simulink model "Base_Map_M_cs"  (R2017b)
settings: Solver=FixedStepDiscrete  StartTime=0.0  StopTime=60  FixedStep=1/100  RelTol=1e-3
PreLoadFcn:
  | mbxruntime.callbacks.PreLoadFcn(bdroot);
  | check_NUTS_defined
  | model_closed = 0;
  | assignin('base',['model_closed_' bdroot],false);
PostLoadFcn:
  | mbxruntime.callbacks.PostLoadFcn(bdroot);
InitFcn:
  | mbxruntime.callbacks.InitFcn(bdroot);
StartFcn:
  | mbxruntime.callbacks.StartFcn(bdroot);
StopFcn:
  | mbxruntime.callbacks.StopFcn(bdroot);;
  | 
model workspace: external: MAT-File Base_Map_M_cs_hws.mat (data not in the file)
undefined symbols (not defined in the file): mbxruntime, tabledata
(part 1 of 3)
CloseFcn:
  | mbxruntime.callbacks.CloseFcn(bdroot);
  | evalin('base',['clear model_closed_' bdroot]);
  | model_closed = 1;
settings Model: Creator=PRESCAN  LastModifiedBy=naveenm
settings DataIOCC: LimitDataPoints=on  SaveFormat=Array  SignalLoggingSaveFormat=ModelDataLogs
settings OptimizationCC: ExpressionDepthLimit=2147483647  InitFltsAndDblsToZero=on  LifeSpan=inf
settings DebuggingCC: SaveWithParameterizedLinksMsg=none  UnderspecifiedInitializationDetection=Classic  MergeDetectMultiDrivingBlocksExec=none  SignalResolutionControl=TryResolveAllWithWarning  MultiTaskDSMMsg=warning  MultiTaskCondExecSysMsg=none  FcnCallInpInsideContextMsg=warning  StateNameClashWarn=warning  SFUnexpectedBacktrackingDiag=warning  SFNoUnconditionalDefaultTransitionDiag=warning  SFExecutionAtInitializationDiag=none
settings HardwareCC: ProdBitPerPointer=32  ProdBitPerSizeT=32  ProdBitPerPtrDiffT=32  ProdLargestAtomicFloat=None  ProdIntDivRoundTo=Undefined  ProdEndianess=Unspecified  ProdWordSize=32  ProdHWDeviceType=32-bit Generic
settings ModelReferenceCC: UpdateModelReferenceTargets=IfOutOfDate  PropagateSignalLabelsOutOfModel=off
settings SFSimCC: SimParseCustomCode=off
settings SFSimCC: SimCustomHeaderCode=|
  | #include "prescan.h"
  | #include "prescan_platform.h"
settings CodeAppCC: StateflowObjectComments=on
settings GRTTargetCC: TargetFcnLib=ansi_tfl_tmw.mat  TargetLangStandard=C89/C90 (ANSI)  GeneratePreprocessorConditionals=Disable all  CombineOutputUpdateFcns=off  GRTInterface=on
settings ConfigComp: CovMetricSettings=dw  CovHtmlReporting=on  CovSaveCumulativeToWorkspaceVar=on  CovSaveSingleToWorkspaceVar=on  CovExternalEMLEnable=off

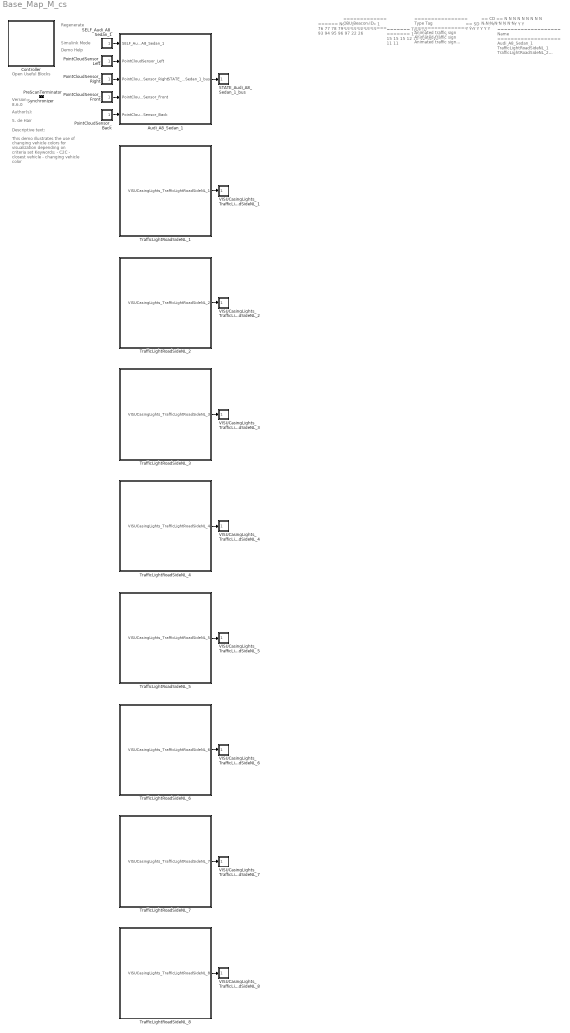
== system Base_Map_M_cs ==
  note: Regenerate
  note: Simulink Mode
  note: Open Useful Blocks
  note: 8.6.0
  note: Version:
  note: Author(s):
  note: S. de Hair
  note: Descriptive text:
  note: This demo illustrates the use of
      | changing vehicle colors for
      | visualization depending on
      | criteria set
      |
      |
      |
      | Keywords:
      |
      | - C2C
      |
      | - closest vehicle
      |
      | - changing vehicle color
  note: Demo Help
  note: ======
      | Num ID
      | ======
      | 1
      | 76
      | 77
      | 78
      | 79
      | 80
      | 81
      | 82
      | 83
      | 91
      | 93
      | 94
      | 95
      | 96
      | 97
      | 22
      | 26
  note: =============
      | OBU-Beacon ID
      | =============
  note: =======
      | Type ID
      | =======
      | 1
      | 15
      | 15
      | 15
      | 15
      | 15
      | 15
      | 15
      | 15
      | 12
      | 12
      | 12
      | 12
      | 12
      | 12
      | 11
      | 11
  note: ================
      | Type Tag
      | ================
      | Car
      | Animated traffic sign
      | Animated traffic sign
      | Animated traffic sign
      | Animated traffic sign
      | Animated traffic sign
      | Animated traffic sign
      | Animated traffic sign
      | Animated traffic sign
      | Building
      | Building
      | Building
      | Building
      | Building
      | Building
      | Road
      | Road
  note: ==
      | SD
      | ==
      | Y
      | Y
      | Y
      | Y
      | Y
      | Y
      | Y
      | Y
      | Y
      | Y
      | Y
      | Y
      | Y
      | Y
      | Y
      | Y
      | Y
  note: ==
      | CD
      | ==
      | N
      | N
      | N
      | N
      | N
      | N
      | N
      | N
      | N
      | N
      | N
      | N
      | N
      | N
      | N
      | N
      | N
  note: ===================
      | Name
      | ===================
      | Audi_A8_Sedan_1
      | TrafficLightRoadSideNL_1
      | TrafficLightRoadSideNL_2
      | TrafficLightRoadSideNL_3
      | TrafficLightRoadSideNL_4
      | TrafficLightRoadSideNL_5
      | TrafficLightRoadSideNL_6
      | TrafficLightRoadSideNL_7
      | TrafficLightRoadSideNL_8
      | HouseOld3_1
      | HouseOld4_1
      | HouseOld5_1
      | School_1
      | OfficeBrownFlat_1
      | OfficeBrownTall2_1
      | StraightRoad_2
      | StraightRoad_5
  Audi_A8_Sedan_1 : Subsystem  Tag=WorldObjectSubSystem  InitFcn=UniqueId = '642';
      mask init:
      | modelPath = GenericModelHelper.getGenericModelFilePath('ModelDepo','Vehicles\Audi_A8\Audi_A8.pgmb','d771622804618130053427da08a6d484');imagePath = GenericModelHelper.getCompilationPicture(modelPath, 'Audi_A8_HighPoly.png');
      mask Display: image(imread(imagePath));color('white');text(0, 0, ' ID=1\n')
  Controller : Subsystem  Description=6E19BCF7C30917F51270F1088431415395D17B111411129AD7F824A4489CC94F  Priority=-1  LoadFcn=load PreScanControllerData  mask(PreScan Simulation Controller){prescanversion='8.6.0', ModelReferencing=off, TimeStep=1/100, ControlMode=0, PreScanExecutionMode=on, ControllerCount=0, ControllerIndex=0, ControllerOptions=''}
      mask prompts: prescanversion "PreScan Version"; ModelReferencing "Use Model Referencing"; TimeStep "Upload Period [s]"; ControlMode "Control Mode"; PreScanExecutionMode "Execution Mode"; ControllerCount "Controller Count"; ControllerIndex "Controller Index"; ControllerOptions "Controller Options"
      mask help:
      | Please do not remove this block from the compilation sheet,
      | as it connects the model to the PreScan environment.
      mask init:
      | model = bdroot(gcb);
      | ExperimentFile = mbxruntime.findExperimentFile(model,true); %relative path
      | 
      | [d1, d2, d3, prescandata] = prescan_Settings();
      | ModelDepo = fullfile(prescandata,'ModelDepo'); 
      | 
      | RTmode = mbxruntime.getRTMode(model);
      | 
      | SimulationMode = get_param(bdroot,'SimulationMode');
      | if strcmp(SimulationMode, 'rapid-accelerator')
      |     SimulationMode = 'external';
      | end
      | TargetName = get_param(bdroot,'SystemTargetFile');
      settings: ModelCloseFcn=assignin('base',['model_closed_' bdroot],true);
      mask Help: eval('openHelp(812)')
      mask Display: image(imread('prescanlogo.ico'))
  PointCloudSensor_Back : Subsystem  Tag=sensor/PointCloudInport  Priority=3  mask(PreScan Source Block: Point Cloud Sensor){}
      mask help: The Point Cloud Sensor provides XYZ positions relative to the sensor
      settings: OpenFcn=open_system([gcb '/Sensor'],'mask')
      mask Help: eval('openHelp(6400)')
      mask Display: image(imread('PointCloudSensorSL.png'))
  PointCloudSensor_Front : Subsystem  Tag=sensor/PointCloudInport  Priority=3  mask(PreScan Source Block: Point Cloud Sensor){}
      mask help: The Point Cloud Sensor provides XYZ positions relative to the sensor
      settings: OpenFcn=open_system([gcb '/Sensor'],'mask')
      mask Help: eval('openHelp(6400)')
      mask Display: image(imread('PointCloudSensorSL.png'))
  PointCloudSensor_Left : Subsystem  Tag=sensor/PointCloudInport  Priority=3  mask(PreScan Source Block: Point Cloud Sensor){}
      mask help: The Point Cloud Sensor provides XYZ positions relative to the sensor
      settings: OpenFcn=open_system([gcb '/Sensor'],'mask')
      mask Help: eval('openHelp(6400)')
      mask Display: image(imread('PointCloudSensorSL.png'))
  PointCloudSensor_Right : Subsystem  Tag=sensor/PointCloudInport  Priority=3  mask(PreScan Source Block: Point Cloud Sensor){}
      mask help: The Point Cloud Sensor provides XYZ positions relative to the sensor
      settings: OpenFcn=open_system([gcb '/Sensor'],'mask')
      mask Help: eval('openHelp(6400)')
      mask Display: image(imread('PointCloudSensorSL.png'))
  PreScanTerminator : Subsystem  Tag=PreScanTerminator  Priority=999  LoadFcn=load PrescanTerminatorData  mask(PreScan Simulation Terminator){TimeStep=1/100}
      mask prompts: TimeStep "Upload Period [s]"
      mask help:
      | Please do not remove this block from the compilation sheet as it
      | connects the model to the PreScan environment.
      mask Help: eval('openHelp(812)')
      mask Display: image(imread('prescanlogo.ico'))
  SELF_Audi_A8_Sedan_1 : Subsystem  Tag=sensor/SelfPort  Priority=3  LoadFcn=load('PreScanSelfSensorData.mat')  mask(PreScan Source Block: SELF){}
      mask help:
      | The SELF port shows (state) information of the actor itself. The outputs are position in the experiment's axis system and the GPS coordinates, and the object's absolute velocity and compass heading.
      |
      | For more information, please click Help.
      settings: OpenFcn=open_system([gcb '/Sensor'],'mask')
      mask Help: eval('openHelp(462)')
      mask Display: image(imread('GPS.png'))
  STATE_Audi_A8_Sedan_1_bus : Subsystem  Tag=actuator/StatePort  Priority=0  LoadFcn=load('PreScanStateActuatorData.mat')  mask(PreScan Sink Block: State){}
      mask help:
      | The Actor State contains a vector signal of size (9x1), containing the following signals:
      |
      | -  Position    	(x,y,z)             	[m]
      | -  Velocity    	(vx,vy,vz)         	[m/s]
      | -  Angles       	(Roll, Pitch, Yaw)	[rad]
      |
      | The Actor state is defined in the global axis system.
      | The state is superponed on the Initial position defined in the GUI.
      |
      | For more information, please click Help.
      settings: OpenFcn=open_system([gcb '/Actuator'],'mask')
      mask Help: eval('openHelp(222)')
      mask Display: image(imread('State.png'))
  Synchronizer : Subsystem  Tag=PreScanSynchronizer  Priority=1  LoadFcn=load PrescanSynchronizeData  mask(PreScan Simulation Core Block){TimeStep=1/100}
      mask prompts: TimeStep "Timestep [s]"
      mask help:
      | Please do not remove this block from the PreScan compilation sheet,
      | as it contains essential configuration parameters for a PreScan simulation.
      settings: DeleteFcn=PreScanBlockDeleteFcn;
      mask Display: image(imread('prescanlogo.ico'))
  TrafficLightRoadSideNL_1 : Subsystem  Tag=WorldObjectSubSystem  InitFcn=UniqueId = '646';
      mask init:
      | imagePath=which('TrafficLightRoadSideNL.jpg');
      mask Display: image(imread(imagePath));color('white');text(0, 0, ' ID=76\n')
  TrafficLightRoadSideNL_2 : Subsystem  Tag=WorldObjectSubSystem  InitFcn=UniqueId = '647';
      mask init:
      | imagePath=which('TrafficLightRoadSideNL.jpg');
      mask Display: image(imread(imagePath));color('white');text(0, 0, ' ID=77\n')
  TrafficLightRoadSideNL_3 : Subsystem  Tag=WorldObjectSubSystem  InitFcn=UniqueId = '649';
      mask init:
      | imagePath=which('TrafficLightRoadSideNL.jpg');
      mask Display: image(imread(imagePath));color('white');text(0, 0, ' ID=78\n')
  TrafficLightRoadSideNL_4 : Subsystem  Tag=WorldObjectSubSystem  InitFcn=UniqueId = '650';
      mask init:
      | imagePath=which('TrafficLightRoadSideNL.jpg');
      mask Display: image(imread(imagePath));color('white');text(0, 0, ' ID=79\n')
  TrafficLightRoadSideNL_5 : Subsystem  Tag=WorldObjectSubSystem  InitFcn=UniqueId = '651';
      mask init:
      | imagePath=which('TrafficLightRoadSideNL.jpg');
      mask Display: image(imread(imagePath));color('white');text(0, 0, ' ID=80\n')
  TrafficLightRoadSideNL_6 : Subsystem  Tag=WorldObjectSubSystem  InitFcn=UniqueId = '652';
      mask init:
      | imagePath=which('TrafficLightRoadSideNL.jpg');
      mask Display: image(imread(imagePath));color('white');text(0, 0, ' ID=81\n')
  TrafficLightRoadSideNL_7 : Subsystem  Tag=WorldObjectSubSystem  InitFcn=UniqueId = '653';
      mask init:
      | imagePath=which('TrafficLightRoadSideNL.jpg');
      mask Display: image(imread(imagePath));color('white');text(0, 0, ' ID=82\n')
  TrafficLightRoadSideNL_8 : Subsystem  Tag=WorldObjectSubSystem  InitFcn=UniqueId = '654';
      mask init:
      | imagePath=which('TrafficLightRoadSideNL.jpg');
      mask Display: image(imread(imagePath));color('white');text(0, 0, ' ID=83\n')
  VISUCasingLights_TrafficLightRoadSideNL_1 : Subsystem  Tag=actuator/VisuCasingLights  Priority=0  mask(PreScan Sink Block: VisuTrafficLight){UniqueID=646, ColorsObjectQuery=, Colors=[]}
      mask prompts: UniqueID "Parent Unique Identifier"; ColorsObjectQuery "Query for Color Object"; Colors "Matrix of colors"
      mask help:
      | The VisuTrafficLight block provides a way to animate traffic lights: switch on and off individual lights.
      |
      | For more information, please click Help.
      settings: OpenFcn=open_system([gcb '/Actuator'],'mask')
      mask Help: eval('openHelp(731)')
      mask Display: image(imread('TrafficLightCasing.png'))
  VISUCasingLights_TrafficLightRoadSideNL_2 : Subsystem  Tag=actuator/VisuCasingLights  Priority=0  mask(PreScan Sink Block: VisuTrafficLight){UniqueID=647, ColorsObjectQuery=, Colors=[]}
      mask prompts: UniqueID "Parent Unique Identifier"; ColorsObjectQuery "Query for Color Object"; Colors "Matrix of colors"
      mask help:
      | The VisuTrafficLight block provides a way to animate traffic lights: switch on and off individual lights.
      |
      | For more information, please click Help.
      settings: OpenFcn=open_system([gcb '/Actuator'],'mask')
      mask Help: eval('openHelp(731)')
      mask Display: image(imread('TrafficLightCasing.png'))
  VISUCasingLights_TrafficLightRoadSideNL_3 : Subsystem  Tag=actuator/VisuCasingLights  Priority=0  mask(PreScan Sink Block: VisuTrafficLight){UniqueID=649, ColorsObjectQuery=, Colors=[]}
      mask prompts: UniqueID "Parent Unique Identifier"; ColorsObjectQuery "Query for Color Object"; Colors "Matrix of colors"
      mask help:
      | The VisuTrafficLight block provides a way to animate traffic lights: switch on and off individual lights.
      |
      | For more information, please click Help.
      settings: OpenFcn=open_system([gcb '/Actuator'],'mask')
      mask Help: eval('openHelp(731)')
      mask Display: image(imread('TrafficLightCasing.png'))
  VISUCasingLights_TrafficLightRoadSideNL_4 : Subsystem  Tag=actuator/VisuCasingLights  Priority=0  mask(PreScan Sink Block: VisuTrafficLight){UniqueID=650, ColorsObjectQuery=, Colors=[]}
      mask prompts: UniqueID "Parent Unique Identifier"; ColorsObjectQuery "Query for Color Object"; Colors "Matrix of colors"
      mask help:
      | The VisuTrafficLight block provides a way to animate traffic lights: switch on and off individual lights.
      |
      | For more information, please click Help.
      settings: OpenFcn=open_system([gcb '/Actuator'],'mask')
      mask Help: eval('openHelp(731)')
      mask Display: image(imread('TrafficLightCasing.png'))
  VISUCasingLights_TrafficLightRoadSideNL_5 : Subsystem  Tag=actuator/VisuCasingLights  Priority=0  mask(PreScan Sink Block: VisuTrafficLight){UniqueID=651, ColorsObjectQuery=, Colors=[]}
      mask prompts: UniqueID "Parent Unique Identifier"; ColorsObjectQuery "Query for Color Object"; Colors "Matrix of colors"
      mask help:
      | The VisuTrafficLight block provides a way to animate traffic lights: switch on and off individual lights.
      |
      | For more information, please click Help.
      settings: OpenFcn=open_system([gcb '/Actuator'],'mask')
      mask Help: eval('openHelp(731)')
      mask Display: image(imread('TrafficLightCasing.png'))
  VISUCasingLights_TrafficLightRoadSideNL_6 : Subsystem  Tag=actuator/VisuCasingLights  Priority=0  mask(PreScan Sink Block: VisuTrafficLight){UniqueID=652, ColorsObjectQuery=, Colors=[]}
      mask prompts: UniqueID "Parent Unique Identifier"; ColorsObjectQuery "Query for Color Object"; Colors "Matrix of colors"
      mask help:
      | The VisuTrafficLight block provides a way to animate traffic lights: switch on and off individual lights.
      |
      | For more information, please click Help.
      settings: OpenFcn=open_system([gcb '/Actuator'],'mask')
      mask Help: eval('openHelp(731)')
      mask Display: image(imread('TrafficLightCasing.png'))
  VISUCasingLights_TrafficLightRoadSideNL_7 : Subsystem  Tag=actuator/VisuCasingLights  Priority=0  mask(PreScan Sink Block: VisuTrafficLight){UniqueID=653, ColorsObjectQuery=, Colors=[]}
      mask prompts: UniqueID "Parent Unique Identifier"; ColorsObjectQuery "Query for Color Object"; Colors "Matrix of colors"
      mask help:
      | The VisuTrafficLight block provides a way to animate traffic lights: switch on and off individual lights.
      |
      | For more information, please click Help.
      settings: OpenFcn=open_system([gcb '/Actuator'],'mask')
      mask Help: eval('openHelp(731)')
      mask Display: image(imread('TrafficLightCasing.png'))
  VISUCasingLights_TrafficLightRoadSideNL_8 : Subsystem  Tag=actuator/VisuCasingLights  Priority=0  mask(PreScan Sink Block: VisuTrafficLight){UniqueID=654, ColorsObjectQuery=, Colors=[]}
      mask prompts: UniqueID "Parent Unique Identifier"; ColorsObjectQuery "Query for Color Object"; Colors "Matrix of colors"
      mask help:
      | The VisuTrafficLight block provides a way to animate traffic lights: switch on and off individual lights.
      |
      | For more information, please click Help.
      settings: OpenFcn=open_system([gcb '/Actuator'],'mask')
      mask Help: eval('openHelp(731)')
      mask Display: image(imread('TrafficLightCasing.png'))
  wires:
  Audi_A8_Sedan_1/1(STATE_Audi_A8_Sedan_1_bus) -> STATE_Audi_A8_Sedan_1_bus/1(STATE_Audi_A8_Sedan_1_bus)
  SELF_Audi_A8_Sedan_1/1(SELF_Audi_A8_Sedan_1) -> Audi_A8_Sedan_1/1(SELF_Audi_A8_Sedan_1)
  PointCloudSensor_Left/1(PointCloudSensor_Left) -> Audi_A8_Sedan_1/2(PointCloudSensor_Left)
  PointCloudSensor_Right/1(PointCloudSensor_Right) -> Audi_A8_Sedan_1/3(PointCloudSensor_Right)
  PointCloudSensor_Front/1(PointCloudSensor_Front) -> Audi_A8_Sedan_1/4(PointCloudSensor_Front)
  PointCloudSensor_Back/1(PointCloudSensor_Back) -> Audi_A8_Sedan_1/5(PointCloudSensor_Back)
  TrafficLightRoadSideNL_1/1(VISUCasingLights_TrafficLightRoadSideNL_1) -> VISUCasingLights_TrafficLightRoadSideNL_1/1(VISUCasingLights_TrafficLightRoadSideNL_1)
  TrafficLightRoadSideNL_2/1(VISUCasingLights_TrafficLightRoadSideNL_2) -> VISUCasingLights_TrafficLightRoadSideNL_2/1(VISUCasingLights_TrafficLightRoadSideNL_2)
  TrafficLightRoadSideNL_3/1(VISUCasingLights_TrafficLightRoadSideNL_3) -> VISUCasingLights_TrafficLightRoadSideNL_3/1(VISUCasingLights_TrafficLightRoadSideNL_3)
  TrafficLightRoadSideNL_4/1(VISUCasingLights_TrafficLightRoadSideNL_4) -> VISUCasingLights_TrafficLightRoadSideNL_4/1(VISUCasingLights_TrafficLightRoadSideNL_4)
  TrafficLightRoadSideNL_5/1(VISUCasingLights_TrafficLightRoadSideNL_5) -> VISUCasingLights_TrafficLightRoadSideNL_5/1(VISUCasingLights_TrafficLightRoadSideNL_5)
  TrafficLightRoadSideNL_6/1(VISUCasingLights_TrafficLightRoadSideNL_6) -> VISUCasingLights_TrafficLightRoadSideNL_6/1(VISUCasingLights_TrafficLightRoadSideNL_6)
  TrafficLightRoadSideNL_7/1(VISUCasingLights_TrafficLightRoadSideNL_7) -> VISUCasingLights_TrafficLightRoadSideNL_7/1(VISUCasingLights_TrafficLightRoadSideNL_7)
  TrafficLightRoadSideNL_8/1(VISUCasingLights_TrafficLightRoadSideNL_8) -> VISUCasingLights_TrafficLightRoadSideNL_8/1(VISUCasingLights_TrafficLightRoadSideNL_8)

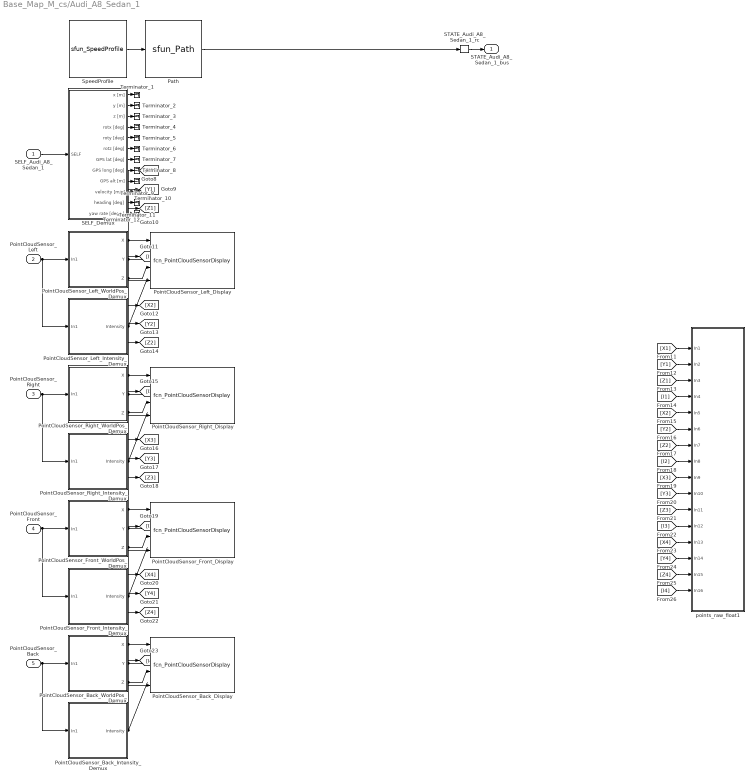
== system Base_Map_M_cs/Audi_A8_Sedan_1 ==
  SELF_Audi_A8_Sedan_1 : Inport  Tag=inport/SelfPort  OutDataTypeStr=Bus: PRESCAN_SELFSENSORDATA  PortDimensions=1  SampleTime=1/100  BusOutputAsStruct=on
  PointCloudSensor_Left : Inport  Tag=inport/PointCloudInport  Port=2  OutDataTypeStr=single  SampleTime=1/1  BusOutputAsStruct=on
  PointCloudSensor_Right : Inport  Tag=inport/PointCloudInport  Port=3  OutDataTypeStr=single  SampleTime=1/1  BusOutputAsStruct=on
  PointCloudSensor_Front : Inport  Tag=inport/PointCloudInport  Port=4  OutDataTypeStr=single  SampleTime=1/1  BusOutputAsStruct=on
  PointCloudSensor_Back : Inport  Tag=inport/PointCloudInport  Port=5  OutDataTypeStr=single  SampleTime=1/1  BusOutputAsStruct=on
  Path : S-Function  Tag=Path  LoadFcn=load('PrescanMotionData.mat')  FunctionName=sfun_Path  Parameters=uniqueID, pathUniqueID, timestep  SFunctionDeploymentMode=off  EnableBusSupport=off  mask(Path){uniqueID=642, pathUniqueID=7771, timestep=1/100}
      mask prompts: uniqueID "Object Unique ID"; pathUniqueID "Path Unique ID"; timestep "MATLAB timestep:"
      mask help:
      | The path block outputs the position along a given trajectory.
      |
      | For more information, please click Help.
      mask Help: eval('openHelp(312)')
      mask Display: image(imread('Path.png'))
  PointCloudSensor_Back_Display : M-S-Function  Tag=PointCloudSensor_Display  FunctionName=fcn_PointCloudSensorDisplay  Parameters=SensorName EnableDisplay FigureHandle EnableIntensity  mask(PreScan Point Cloud Display Block){SensorName=PointCloudSensor_Back, EnableDisplay=off, FigureHandle=64204, EnableIntensity=on}
      mask prompts: SensorName "User Specified: Title of Display"; EnableDisplay "Active"; FigureHandle "Unique Handle"; EnableIntensity "Visualize Intensity"
      mask help: This block displays world position (and intensity) output of a PreScan point cloud sensor.
      mask init:
      | if EnableDisplay
      |     EnableString='';
      |     EnableColor='gray';
      | else
      |     EnableString='INACTIVE';
      |     EnableColor='red';
      | end
      settings: DeleteFcn=PreScanBlockDeleteFcn;  ModelCloseFcn=fcn_ImageDisplay_ModelCloseFcn
      mask Help: eval('openHelp(6400)')
      mask Display:
      | color(EnableColor);
      | fprintf('%s\n PointCloud Display:\n %s',EnableString,SensorName)
      | port_label('input',1,'X')
      | port_label('input',2,'Y')
      | port_label('input',3,'Z')
      | 
      | if EnableIntensity
      |     port_label('input',4,'I')
      | end
  PointCloudSensor_Back_Intensity_Demux : Subsystem  Tag=demux/PCS/Intensity  mask{SensorName=PointCloudSensor_Back, offset=480, hres=160, vres=40}
      mask prompts: SensorName "Sensor Name"; offset "Data Start"; hres "Horizontal Resolution"; vres "Vertical Resolution"
      mask Help: eval('openHelp(6400)')
      mask Display:
      | fprintf('Point Cloud:\n Data\n %s \n %d x %d px',SensorName,hres,vres)
      | port_label('output',1,'Intensity')
  PointCloudSensor_Back_WorldPos_Demux : Subsystem  Tag=demux/PCS/WorldPos  mask{SensorName=PointCloudSensor_Back, offset=0, hres=160, vres=40}
      mask prompts: SensorName "Sensor Name"; offset "Data Start"; hres "Horizontal Resolution"; vres "Vertical Resolution"
      mask Help: eval('openHelp(6400)')
      mask Display:
      | fprintf('Point Cloud:\n Data\n %s \n %d x %d px',SensorName,hres,vres)
      | port_label('output',1,'X')
      | port_label('output',2,'Y')
      | port_label('output',3,'Z')
  PointCloudSensor_Front_Display : M-S-Function  Tag=PointCloudSensor_Display  FunctionName=fcn_PointCloudSensorDisplay  Parameters=SensorName EnableDisplay FigureHandle EnableIntensity  mask(PreScan Point Cloud Display Block){SensorName=PointCloudSensor_Front, EnableDisplay=off, FigureHandle=64203, EnableIntensity=on}
      mask prompts: SensorName "User Specified: Title of Display"; EnableDisplay "Active"; FigureHandle "Unique Handle"; EnableIntensity "Visualize Intensity"
      mask help: This block displays world position (and intensity) output of a PreScan point cloud sensor.
      mask init:
      | if EnableDisplay
      |     EnableString='';
      |     EnableColor='gray';
      | else
      |     EnableString='INACTIVE';
      |     EnableColor='red';
      | end
      settings: DeleteFcn=PreScanBlockDeleteFcn;  ModelCloseFcn=fcn_ImageDisplay_ModelCloseFcn
      mask Help: eval('openHelp(6400)')
      mask Display:
      | color(EnableColor);
      | fprintf('%s\n PointCloud Display:\n %s',EnableString,SensorName)
      | port_label('input',1,'X')
      | port_label('input',2,'Y')
      | port_label('input',3,'Z')
      | 
      | if EnableIntensity
      |     port_label('input',4,'I')
      | end
  PointCloudSensor_Front_Intensity_Demux : Subsystem  Tag=demux/PCS/Intensity  mask{SensorName=PointCloudSensor_Front, offset=480, hres=160, vres=40}
      mask prompts: SensorName "Sensor Name"; offset "Data Start"; hres "Horizontal Resolution"; vres "Vertical Resolution"
      mask Help: eval('openHelp(6400)')
      mask Display:
      | fprintf('Point Cloud:\n Data\n %s \n %d x %d px',SensorName,hres,vres)
      | port_label('output',1,'Intensity')
  PointCloudSensor_Front_WorldPos_Demux : Subsystem  Tag=demux/PCS/WorldPos  mask{SensorName=PointCloudSensor_Front, offset=0, hres=160, vres=40}
      mask prompts: SensorName "Sensor Name"; offset "Data Start"; hres "Horizontal Resolution"; vres "Vertical Resolution"
      mask Help: eval('openHelp(6400)')
      mask Display:
      | fprintf('Point Cloud:\n Data\n %s \n %d x %d px',SensorName,hres,vres)
      | port_label('output',1,'X')
      | port_label('output',2,'Y')
      | port_label('output',3,'Z')
  PointCloudSensor_Left_Display : M-S-Function  Tag=PointCloudSensor_Display  FunctionName=fcn_PointCloudSensorDisplay  Parameters=SensorName EnableDisplay FigureHandle EnableIntensity  mask(PreScan Point Cloud Display Block){SensorName=PointCloudSensor_Left, EnableDisplay=off, FigureHandle=64201, EnableIntensity=on}
      mask prompts: SensorName "User Specified: Title of Display"; EnableDisplay "Active"; FigureHandle "Unique Handle"; EnableIntensity "Visualize Intensity"
      mask help: This block displays world position (and intensity) output of a PreScan point cloud sensor.
      mask init:
      | if EnableDisplay
      |     EnableString='';
      |     EnableColor='gray';
      | else
      |     EnableString='INACTIVE';
      |     EnableColor='red';
      | end
      settings: DeleteFcn=PreScanBlockDeleteFcn;  ModelCloseFcn=fcn_ImageDisplay_ModelCloseFcn
      mask Help: eval('openHelp(6400)')
      mask Display:
      | color(EnableColor);
      | fprintf('%s\n PointCloud Display:\n %s',EnableString,SensorName)
      | port_label('input',1,'X')
      | port_label('input',2,'Y')
      | port_label('input',3,'Z')
      | 
      | if EnableIntensity
      |     port_label('input',4,'I')
      | end
  PointCloudSensor_Left_Intensity_Demux : Subsystem  Tag=demux/PCS/Intensity  mask{SensorName=PointCloudSensor_Left, offset=480, hres=160, vres=40}
      mask prompts: SensorName "Sensor Name"; offset "Data Start"; hres "Horizontal Resolution"; vres "Vertical Resolution"
      mask Help: eval('openHelp(6400)')
      mask Display:
      | fprintf('Point Cloud:\n Data\n %s \n %d x %d px',SensorName,hres,vres)
      | port_label('output',1,'Intensity')
  PointCloudSensor_Left_WorldPos_Demux : Subsystem  Tag=demux/PCS/WorldPos  mask{SensorName=PointCloudSensor_Left, offset=0, hres=160, vres=40}
      mask prompts: SensorName "Sensor Name"; offset "Data Start"; hres "Horizontal Resolution"; vres "Vertical Resolution"
      mask Help: eval('openHelp(6400)')
      mask Display:
      | fprintf('Point Cloud:\n Data\n %s \n %d x %d px',SensorName,hres,vres)
      | port_label('output',1,'X')
      | port_label('output',2,'Y')
      | port_label('output',3,'Z')
  PointCloudSensor_Right_Display : M-S-Function  Tag=PointCloudSensor_Display  FunctionName=fcn_PointCloudSensorDisplay  Parameters=SensorName EnableDisplay FigureHandle EnableIntensity  mask(PreScan Point Cloud Display Block){SensorName=PointCloudSensor_Right, EnableDisplay=off, FigureHandle=64202, EnableIntensity=on}
      mask prompts: SensorName "User Specified: Title of Display"; EnableDisplay "Active"; FigureHandle "Unique Handle"; EnableIntensity "Visualize Intensity"
      mask help: This block displays world position (and intensity) output of a PreScan point cloud sensor.
      mask init:
      | if EnableDisplay
      |     EnableString='';
      |     EnableColor='gray';
      | else
      |     EnableString='INACTIVE';
      |     EnableColor='red';
      | end
      settings: DeleteFcn=PreScanBlockDeleteFcn;  ModelCloseFcn=fcn_ImageDisplay_ModelCloseFcn
      mask Help: eval('openHelp(6400)')
      mask Display:
      | color(EnableColor);
      | fprintf('%s\n PointCloud Display:\n %s',EnableString,SensorName)
      | port_label('input',1,'X')
      | port_label('input',2,'Y')
      | port_label('input',3,'Z')
      | 
      | if EnableIntensity
      |     port_label('input',4,'I')
      | end
  PointCloudSensor_Right_Intensity_Demux : Subsystem  Tag=demux/PCS/Intensity  mask{SensorName=PointCloudSensor_Right, offset=480, hres=160, vres=40}
      mask prompts: SensorName "Sensor Name"; offset "Data Start"; hres "Horizontal Resolution"; vres "Vertical Resolution"
      mask Help: eval('openHelp(6400)')
      mask Display:
      | fprintf('Point Cloud:\n Data\n %s \n %d x %d px',SensorName,hres,vres)
      | port_label('output',1,'Intensity')
  PointCloudSensor_Right_WorldPos_Demux : Subsystem  Tag=demux/PCS/WorldPos  mask{SensorName=PointCloudSensor_Right, offset=0, hres=160, vres=40}
      mask prompts: SensorName "Sensor Name"; offset "Data Start"; hres "Horizontal Resolution"; vres "Vertical Resolution"
      mask Help: eval('openHelp(6400)')
      mask Display:
      | fprintf('Point Cloud:\n Data\n %s \n %d x %d px',SensorName,hres,vres)
      | port_label('output',1,'X')
      | port_label('output',2,'Y')
      | port_label('output',3,'Z')
  SELF_Demux : Subsystem  Tag=demux/SelfPort  mask(PreScan Demux Block:){}
      mask help:
      | The SELF port shows (state) information of the actor itself. The outputs are position in the experiment's axis system and the GPS coordinates, and the object's absolute velocity and compass heading.
      |
      | For more information, please click Help.
      settings: DeleteFcn=PreScanBlockDeleteFcn;
      mask Help: eval('openHelp(462)')
      mask Display:
      | port_label('output',1,'x [m]')
      | port_label('output',2,'y [m]')
      | port_label('output',3,'z [m]','texmode','on')
      | port_label('output',4,'Rotx [deg]','texmode','on')
      | port_label('output',5,'Roty [deg]','texmode','on')
      | port_label('output',6,'Rotz [deg]','texmode','on')
      | port_label('output',7,'GPS lat [deg]','texmode','on')
      | port_label('output',8,'GPS long [deg]','texmode','on')
      | port_label('output',9,'GPS alt [m]','texmode','on')
      | port_label('output',10,'Velocity [m/s]')
      | port_label('output',11,'Heading [deg]')
      | port_label('output',12,'Yaw rate [deg/s]')
  STATE_Audi_A8_Sedan_1_rc : RateTransition  Tag=mux_rc/StatePort  OutPortSampleTimeOpt=Inherit
  SpeedProfile : S-Function  Tag=SpeedProfile  LoadFcn=load('PrescanMotionData.mat')  FunctionName=sfun_SpeedProfile  Parameters=speedProfileUniqueID, timestep  SFunctionDeploymentMode=off  EnableBusSupport=off  mask(SpeedProfile){speedProfileUniqueID=7772, timestep=1/100}
      mask prompts: speedProfileUniqueID "Speed Profile Unique ID"; timestep "MATLAB timestep:"
      mask help:
      | The speed profile block outputs the travelled distance, velocities and acceleration along a given path.
      |
      | For more information, please click Help.
      mask Help: eval('openHelp(312)')
      mask Display: image(imread('SpeedProfile.png'))
  Terminator_{1..12} (12 alike) : Terminator
  points_raw_float1 : Subsystem
  STATE_Audi_A8_Sedan_1_bus : Outport  Tag=outport/StatePort  OutDataTypeStr=Bus: PRESCAN_STATEACTUATORDATA  PortDimensions=1  SampleTime=1/100
  wires:
  [X1] -> points_raw_float1/1(In1)
  [Y1] -> points_raw_float1/2(In2)
  [Z1] -> points_raw_float1/3(In3)
  [I1] -> points_raw_float1/4(In4)
  [I2] -> points_raw_float1/8(In8)
  [Z2] -> points_raw_float1/7(In7)
  [Y2] -> points_raw_float1/6(In6)
  [X2] -> points_raw_float1/5(In5)
  [I3] -> points_raw_float1/12(In12)
  [Z3] -> points_raw_float1/11(In11)
  [Y3] -> points_raw_float1/10(In10)
  [X3] -> points_raw_float1/9(In9)
  [I4] -> points_raw_float1/16(In16)
  [Z4] -> points_raw_float1/15(In15)
  [Y4] -> points_raw_float1/14(In14)
  [X4] -> points_raw_float1/13(In13)
  PointCloudSensor_Left_WorldPos_Demux/1(X) -> [X1], PointCloudSensor_Left_Display/1
  PointCloudSensor_Left_WorldPos_Demux/2(Y) -> [Y1], PointCloudSensor_Left_Display/2
  PointCloudSensor_Left_WorldPos_Demux/3(Z) -> [Z1], PointCloudSensor_Left_Display/3
  PointCloudSensor_Left_Intensity_Demux/1(Intensity) -> [I1], PointCloudSensor_Left_Display/4
  PointCloudSensor_Right_WorldPos_Demux/1(X) -> [X2], PointCloudSensor_Right_Display/1
  PointCloudSensor_Right_WorldPos_Demux/2(Y) -> [Y2], PointCloudSensor_Right_Display/2
  PointCloudSensor_Right_WorldPos_Demux/3(Z) -> [Z2], PointCloudSensor_Right_Display/3
  PointCloudSensor_Right_Intensity_Demux/1(Intensity) -> [I2], PointCloudSensor_Right_Display/4
  PointCloudSensor_Front_WorldPos_Demux/1(X) -> [X3], PointCloudSensor_Front_Display/1
  PointCloudSensor_Front_WorldPos_Demux/2(Y) -> [Y3], PointCloudSensor_Front_Display/2
  PointCloudSensor_Front_WorldPos_Demux/3(Z) -> [Z3], PointCloudSensor_Front_Display/3
  PointCloudSensor_Front_Intensity_Demux/1(Intensity) -> [I3], PointCloudSensor_Front_Display/4
  PointCloudSensor_Back_WorldPos_Demux/1(X) -> [X4], PointCloudSensor_Back_Display/1
  PointCloudSensor_Back_WorldPos_Demux/2(Y) -> [Y4], PointCloudSensor_Back_Display/2
  PointCloudSensor_Back_WorldPos_Demux/3(Z) -> [Z4], PointCloudSensor_Back_Display/3
  PointCloudSensor_Back_Intensity_Demux/1(Intensity) -> [I4], PointCloudSensor_Back_Display/4
  STATE_Audi_A8_Sedan_1_rc/1 -> STATE_Audi_A8_Sedan_1_bus/1
  SpeedProfile/1 -> Path/1
  Path/1 -> STATE_Audi_A8_Sedan_1_rc/1
  SELF_Audi_A8_Sedan_1/1 -> SELF_Demux/1(SELF)
  PointCloudSensor_Left/1 -> PointCloudSensor_Left_WorldPos_Demux/1(In1), PointCloudSensor_Left_Intensity_Demux/1(In1)
  PointCloudSensor_Right/1 -> PointCloudSensor_Right_WorldPos_Demux/1(In1), PointCloudSensor_Right_Intensity_Demux/1(In1)
  PointCloudSensor_Front/1 -> PointCloudSensor_Front_WorldPos_Demux/1(In1), PointCloudSensor_Front_Intensity_Demux/1(In1)
  PointCloudSensor_Back/1 -> PointCloudSensor_Back_WorldPos_Demux/1(In1), PointCloudSensor_Back_Intensity_Demux/1(In1)
  SELF_Demux/1(x [m]) -> Terminator_1/1
  SELF_Demux/2(y [m]) -> Terminator_2/1
  SELF_Demux/3(z [m]) -> Terminator_3/1
  SELF_Demux/4(rotx [deg]) -> Terminator_4/1
  SELF_Demux/5(roty [deg]) -> Terminator_5/1
  SELF_Demux/6(rotz [deg]) -> Terminator_6/1
  SELF_Demux/7(GPS lat [deg]) -> Terminator_7/1
  SELF_Demux/8(GPS long [deg]) -> Terminator_8/1
  SELF_Demux/9(GPS alt [m]) -> Terminator_9/1
  SELF_Demux/10(velocity [m/s]) -> Terminator_10/1
  SELF_Demux/11(heading [deg]) -> Terminator_11/1
  SELF_Demux/12(yaw rate [deg/s]) -> Terminator_12/1

== system Base_Map_M_cs/Controller ==
  Terminator : Terminator
  sfun_Controller : S-Function  FunctionName=sfun_Controller  Parameters=SParameter1, SParameter2, SParameter3, SParameter4, SParameter5, SParameter6, SParameter7, SParameter8, SParameter9, SParameter10, SampleTime  SFunctionDeploymentMode=off  EnableBusSupport=off  mask(Legacy Function){SFunctionSpec=void prescan_outputFcn(void** work1, PRESCAN_CONTROLLERDATA y1[1]), SParameter1=uint8([ExperimentFile 0]), SParameter2=uint8([ModelDepo 0]), SParameter3=uint8([ControllerOptions 0]), SParameter4=RTmode, SParameter5=PreScanExecutionMode, SParameter6=ControlMode, SParameter7=ControllerCount, SParameter8=ControllerIndex, SParameter9=uint8([SimulationMode 0]), SParameter10=uint8([TargetName 0]), SampleTime=TimeStep, ShowSpec=on}
      mask prompts: SParameter1 "P1:"; SParameter2 "P2:"; SParameter3 "P3:"; SParameter4 "P4:"; SParameter5 "P5:"; SParameter6 "P6:"; SParameter7 "P7:"; SParameter8 "P8:"; SParameter9 "P9:"; SParameter10 "P10:"; SampleTime "Sample time (-1 for inherited):"; ShowSpec "Display function specification"
      mask help:
      | This block allows you to call the legacy functions specified by the following Legacy Code Tool definition:
      | def.SFunctionName = 'sfun_Controller';
      | def.OutputFcnSpec = 'void prescan_outputFcn(void** work1, PRESCAN_CONTROLLERDATA y1[1])';
      | def.StartFcnSpec = 'void prescan_startFcn(void ** work1, uint8 p1[], uint8 p2[], uint8 p3[], double p4, double p5, double p6, double p7, double p8, uint8 p9[], uint8 p10[])';
      | def.TerminateFcnSpec = 'void prescan_terminateFcn(void** work1)';
      | def.HeaderFiles = {'prescan_controller_data.h', 'prescan_SFunLibrary.h', 'prescan_CreateLogHandler.h', 'prescan_CreateErrorHandler.h', 'prescan_modify.h', 'ModuleDLL.h'};
      | def.SourceFiles = {'prescan_MexLogHandler.c', 'prescan_SimStructErrorHandler.c', 'prescan_LogHandler.c', 'prescan_ErrorHandler.c', 'prescan_Modify.c'};
      | def.HostLibFiles = {'sensorinterfaced.lib'};
      | def.TargetLibFiles = {'sensorinterfaced.so'};
      | def.IncPaths = {'.', 'C:\projects\prescan\rt_vislibrary\vis\..\pimp\include\sensors\InterfaceRTW'};
      | def.SrcPaths = {'C:\projects\prescan\rt_vislibrary\vis\..\pimp\include\sensors\InterfaceRTW', 'C:\projects\prescan\rt_vislibrary\vis\..\pimp\include\sensors\InterfaceRTW\ccurrt'};
      | def.LibPaths = {'C:\\projects\\prescan\\vislibrary_build\lib'};
      | def.SampleTime = 'parameterized';
      mask Help: <p>This block was generated automatically by the Legacy Code Tool. For detailed help on this tool, call<a href="matlab:legacy_code('help')"> legacy_code('help')</a>.</p>
      mask Callback ShowSpec:
      | if strcmp(get_param(gcbh, 'ShowSpec'), 'on')
      |   set_param(gcbh, 'MaskDisplay', sprintf('fprintf(''%s'');', get_param(gcbh, 'SFunctionSpec')));
      | else
      |   set_param(gcbh, 'MaskDisplay', sprintf('fprintf(''%s'');', get_param(gcbh, 'FunctionName')));
      | end
      mask Display: fprintf('void prescan_outputFcn(void** work1, PRESCAN_CONTROLLERDATA y1[1])');
  wires:
  sfun_Controller/1 -> Terminator/1

== system Base_Map_M_cs/PointCloudSensor_Back ==
  Sensor : S-Function  FunctionName=sfun_PCS  Parameters=sensorID, dataWidth, dataHeight, numChannels, dataType, timestep  SFunctionDeploymentMode=off  EnableBusSupport=off  mask(PreScan Source Block: Point Cloud Sensor){sensorID=1408, dataWidth=40, dataHeight=640, numChannels=4, dataType=0, timestep=1/1}
      mask prompts: sensorID "Sensor ID"; dataWidth "Data Width"; dataHeight "Data Height"; numChannels "Channel Count"; dataType "Data Type"; timestep "MATLAB timestep:"
      mask help: The Point Cloud Sensor provides XYZ positions relative to the sensor
      mask Help: eval('openHelp(6400)')
      mask Display: image(imread('PointCloudSensorSL.png'))
  PointCloudSensor_Back : Outport  Tag=outport/PointCloudInport  OutDataTypeStr=single  SampleTime=1/1
  wires:
  Sensor/1 -> PointCloudSensor_Back/1

== system Base_Map_M_cs/PointCloudSensor_Front ==
  Sensor : S-Function  FunctionName=sfun_PCS  Parameters=sensorID, dataWidth, dataHeight, numChannels, dataType, timestep  SFunctionDeploymentMode=off  EnableBusSupport=off  mask(PreScan Source Block: Point Cloud Sensor){sensorID=1406, dataWidth=40, dataHeight=640, numChannels=4, dataType=0, timestep=1/1}
      mask prompts: sensorID "Sensor ID"; dataWidth "Data Width"; dataHeight "Data Height"; numChannels "Channel Count"; dataType "Data Type"; timestep "MATLAB timestep:"
      mask help: The Point Cloud Sensor provides XYZ positions relative to the sensor
      mask Help: eval('openHelp(6400)')
      mask Display: image(imread('PointCloudSensorSL.png'))
  PointCloudSensor_Front : Outport  Tag=outport/PointCloudInport  OutDataTypeStr=single  SampleTime=1/1
  wires:
  Sensor/1 -> PointCloudSensor_Front/1

== system Base_Map_M_cs/PointCloudSensor_Left ==
  Sensor : S-Function  FunctionName=sfun_PCS  Parameters=sensorID, dataWidth, dataHeight, numChannels, dataType, timestep  SFunctionDeploymentMode=off  EnableBusSupport=off  mask(PreScan Source Block: Point Cloud Sensor){sensorID=1401, dataWidth=40, dataHeight=640, numChannels=4, dataType=0, timestep=1/1}
      mask prompts: sensorID "Sensor ID"; dataWidth "Data Width"; dataHeight "Data Height"; numChannels "Channel Count"; dataType "Data Type"; timestep "MATLAB timestep:"
      mask help: The Point Cloud Sensor provides XYZ positions relative to the sensor
      mask Help: eval('openHelp(6400)')
      mask Display: image(imread('PointCloudSensorSL.png'))
  PointCloudSensor_Left : Outport  Tag=outport/PointCloudInport  OutDataTypeStr=single  SampleTime=1/1
  wires:
  Sensor/1 -> PointCloudSensor_Left/1

== system Base_Map_M_cs/PointCloudSensor_Right ==
  Sensor : S-Function  FunctionName=sfun_PCS  Parameters=sensorID, dataWidth, dataHeight, numChannels, dataType, timestep  SFunctionDeploymentMode=off  EnableBusSupport=off  mask(PreScan Source Block: Point Cloud Sensor){sensorID=1402, dataWidth=40, dataHeight=640, numChannels=4, dataType=0, timestep=1/1}
      mask prompts: sensorID "Sensor ID"; dataWidth "Data Width"; dataHeight "Data Height"; numChannels "Channel Count"; dataType "Data Type"; timestep "MATLAB timestep:"
      mask help: The Point Cloud Sensor provides XYZ positions relative to the sensor
      mask Help: eval('openHelp(6400)')
      mask Display: image(imread('PointCloudSensorSL.png'))
  PointCloudSensor_Right : Outport  Tag=outport/PointCloudInport  OutDataTypeStr=single  SampleTime=1/1
  wires:
  Sensor/1 -> PointCloudSensor_Right/1

== system Base_Map_M_cs/PreScanTerminator ==
  Terminator : Terminator
  sfun_Terminator : S-Function  FunctionName=sfun_Terminator  Parameters=SampleTime  SFunctionDeploymentMode=off  EnableBusSupport=off  mask(Legacy Function){SFunctionSpec=void prescan_terminator_outputFcn(void ** work1, PRESCAN_TERMINATORDATA y1[1]), SampleTime=TimeStep, ShowSpec=on}
      mask prompts: SampleTime "Sample time (-1 for inherited):"; ShowSpec "Display function specification"
      mask help:
      | This block allows you to call the legacy functions specified by the following Legacy Code Tool definition:
      | def.SFunctionName = 'sfun_Terminator';
      | def.OutputFcnSpec = 'void prescan_terminator_outputFcn(void ** work1, PRESCAN_TERMINATORDATA y1[1])';
      | def.StartFcnSpec = 'void prescan_terminator_startFcn(void ** work1)';
      | def.TerminateFcnSpec = 'void prescan_terminator_terminateFcn(void ** work1)';
      | def.HeaderFiles = {'prescan_terminator_data.h'};
      | def.HostLibFiles = {'sensorinterfaced.lib'};
      | def.IncPaths = {'src', 'C:\prescandev\vislibrary\vis\..\pimp\include\sensors\InterfaceRTW'};
      | def.SrcPaths = {'src'};
      | def.LibPaths = {'C:\\prescandev\\vislibrary_build\lib'};
      | def.SampleTime = 'parameterized';
      | def.Options.language = 'C';
      mask Help: <p>This block was generated automatically by the Legacy Code Tool. For detailed help on this tool, call<a href="matlab:legacy_code('help')"> legacy_code('help')</a>.</p>
      mask Callback ShowSpec:
      | if strcmp(get_param(gcbh, 'ShowSpec'), 'on')
      |   set_param(gcbh, 'MaskDisplay', sprintf('fprintf(''%s'');', get_param(gcbh, 'SFunctionSpec')));
      | else
      |   set_param(gcbh, 'MaskDisplay', sprintf('fprintf(''%s'');', get_param(gcbh, 'FunctionName')));
      | end
      mask Display: fprintf('void prescan_terminator_outputFcn(void ** work1, PRESCAN_TERMINATORDATA y1[1])');
  wires:
  sfun_Terminator/1 -> Terminator/1

== system Base_Map_M_cs/SELF_Audi_A8_Sedan_1 ==
  Sensor : S-Function  FunctionName=sfun_SelfSensor  Parameters=UniqueID, TimeStep  SFunctionDeploymentMode=off  EnableBusSupport=off  mask(PreScan Source Block: SELF){UniqueID=642, TimeStep=1/100}
      mask prompts: UniqueID "Auto-Assigned: Unique ID"; TimeStep "Auto-Assigned: Upload Period [s]"
      mask help:
      | The SELF port shows (state) information of the actor itself. The outputs are position in the experiment's axis system and the GPS coordinates, and the object's absolute velocity and compass heading.
      |
      | For more information, please click Help.
      mask Help: eval('openHelp(462)')
      mask Display: image(imread('GPS.png'))
  SELF_Audi_A8_Sedan_1 : Outport  Tag=outport/SelfPort  OutDataTypeStr=Bus: PRESCAN_SELFSENSORDATA  PortDimensions=1  SampleTime=1/100
  wires:
  Sensor/1 -> SELF_Audi_A8_Sedan_1/1

== system Base_Map_M_cs/STATE_Audi_A8_Sedan_1_bus ==
  STATE_Audi_A8_Sedan_1_bus : Inport  Tag=inport/StatePort  OutDataTypeStr=Bus: PRESCAN_STATEACTUATORDATA  PortDimensions=1  SampleTime=1/100  BusOutputAsStruct=on
  Actuator : S-Function  FunctionName=sfun_StateActuator  Parameters=UniqueID, TimeStep  SFunctionDeploymentMode=off  EnableBusSupport=off  mask(PreScan Sink Block: State){UniqueID=642, TimeStep=1/100}
      mask prompts: UniqueID "Auto-Assigned: Unique ID"; TimeStep "Auto-Assigned: Upload Period [s]"
      mask help:
      | The Actor State contains a vector signal of size (9x1), containing the following signals:
      |
      | -  Position    	(x,y,z)             	[m]
      | -  Velocity    	(vx,vy,vz)         	[m/s]
      | -  Angles       	(Roll, Pitch, Yaw)	[rad]
      |
      | The Actor state is defined in the global axis system.
      | The state is superponed on the Initial position defined in the GUI.
      |
      | For more information, please click Help.
      mask Help: eval('openHelp(222)')
      mask Display: image(imread('State.png'))
  wires:
  STATE_Audi_A8_Sedan_1_bus/1 -> Actuator/1

== system Base_Map_M_cs/Synchronizer ==
  Bus Selector1 : BusSelector  OutputSignals=FederateStopped
  Stop Simulation : Stop
  sfun_Synchronizer : S-Function  FunctionName=sfun_Synchronizer  Parameters=SampleTime  SFunctionDeploymentMode=off  EnableBusSupport=off  mask(Legacy Function){SFunctionSpec=void prescan_synchronizer_outputFcn(void ** work1, PRESCAN_SYNCHRONIZEDATA y1[1]), SampleTime=TimeStep, ShowSpec=on}
      mask prompts: SampleTime "Sample time (-1 for inherited):"; ShowSpec "Display function specification"
      mask help:
      | This block allows you to call the legacy functions specified by the following Legacy Code Tool definition:
      | def.SFunctionName = 'sfun_Synchronizer';
      | def.OutputFcnSpec = 'void prescan_synchronizer_outputFcn(void ** work1, PRESCAN_SYNCHRONIZEDATA y1[1])';
      | def.StartFcnSpec = 'void prescan_synchronizer_startFcn(void ** work1)';
      | def.TerminateFcnSpec = 'void prescan_synchronizer_terminateFcn(void ** work1)';
      | def.HeaderFiles = {'prescan_synchronizer_data.h'};
      | def.HostLibFiles = {'sensorinterfaced.lib'};
      | def.IncPaths = {'src', 'C:\prescandev\vislibrary\vis\..\pimp\include\sensors\InterfaceRTW'};
      | def.SrcPaths = {'src'};
      | def.LibPaths = {'C:\\prescandev\\vislibrary_build\lib'};
      | def.SampleTime = 'parameterized';
      | def.Options.language = 'C';
      mask Help: <p>This block was generated automatically by the Legacy Code Tool. For detailed help on this tool, call<a href="matlab:legacy_code('help')"> legacy_code('help')</a>.</p>
      mask Callback ShowSpec:
      | if strcmp(get_param(gcbh, 'ShowSpec'), 'on')
      |   set_param(gcbh, 'MaskDisplay', sprintf('fprintf(''%s'');', get_param(gcbh, 'SFunctionSpec')));
      | else
      |   set_param(gcbh, 'MaskDisplay', sprintf('fprintf(''%s'');', get_param(gcbh, 'FunctionName')));
      | end
      mask Display: fprintf('void prescan_synchronizer_outputFcn(void ** work1, PRESCAN_SYNCHRONIZEDATA y1[1])');
  wires:
  Bus Selector1/1 -> Stop Simulation/1  "<FederateStopped>"
  sfun_Synchronizer/1 -> Bus Selector1/1

== system Base_Map_M_cs/TrafficLightRoadSideNL_1 ==
  Ground_1 : Ground
  Ground_2 : Ground
  Ground_3 : Ground
  VISUCasingLights_Mux : Subsystem  Tag=mux/VisuCasingLights  mask(PreScan User Interface: VisuTrafficLight){}
      mask help:
      | The VisuTrafficLight block provides a way to animate traffic lights: switch on and off individual lights.
      |
      | For more information, please click Help.
      mask Help: eval('openHelp(731)')
  VISUCasingLights_TrafficLightRoadSideNL_1 : Outport  Tag=outport/VisuCasingLights  SampleTime=1/100
  wires:
  VISUCasingLights_Mux/1(VISUCasingLights_TrafficLightRoadSideNL_1) -> VISUCasingLights_TrafficLightRoadSideNL_1/1
  Ground_1/1 -> VISUCasingLights_Mux/1(Green [-])
  Ground_2/1 -> VISUCasingLights_Mux/2(Orange [-])
  Ground_3/1 -> VISUCasingLights_Mux/3(Red [-])

== system Base_Map_M_cs/TrafficLightRoadSideNL_2 ==
  Ground_1 : Ground
  Ground_2 : Ground
  Ground_3 : Ground
  VISUCasingLights_Mux : Subsystem  Tag=mux/VisuCasingLights  mask(PreScan User Interface: VisuTrafficLight){}
      mask help:
      | The VisuTrafficLight block provides a way to animate traffic lights: switch on and off individual lights.
      |
      | For more information, please click Help.
      mask Help: eval('openHelp(731)')
  VISUCasingLights_TrafficLightRoadSideNL_2 : Outport  Tag=outport/VisuCasingLights  SampleTime=1/100
  wires:
  VISUCasingLights_Mux/1(VISUCasingLights_TrafficLightRoadSideNL_2) -> VISUCasingLights_TrafficLightRoadSideNL_2/1
  Ground_1/1 -> VISUCasingLights_Mux/1(Green [-])
  Ground_2/1 -> VISUCasingLights_Mux/2(Orange [-])
  Ground_3/1 -> VISUCasingLights_Mux/3(Red [-])

== system Base_Map_M_cs/TrafficLightRoadSideNL_3 ==
  Ground_1 : Ground
  Ground_2 : Ground
  Ground_3 : Ground
  VISUCasingLights_Mux : Subsystem  Tag=mux/VisuCasingLights  mask(PreScan User Interface: VisuTrafficLight){}
      mask help:
      | The VisuTrafficLight block provides a way to animate traffic lights: switch on and off individual lights.
      |
      | For more information, please click Help.
      mask Help: eval('openHelp(731)')
  VISUCasingLights_TrafficLightRoadSideNL_3 : Outport  Tag=outport/VisuCasingLights  SampleTime=1/100
  wires:
  VISUCasingLights_Mux/1(VISUCasingLights_TrafficLightRoadSideNL_3) -> VISUCasingLights_TrafficLightRoadSideNL_3/1
  Ground_1/1 -> VISUCasingLights_Mux/1(Green [-])
  Ground_2/1 -> VISUCasingLights_Mux/2(Orange [-])
  Ground_3/1 -> VISUCasingLights_Mux/3(Red [-])

== system Base_Map_M_cs/TrafficLightRoadSideNL_4 ==
  Ground_1 : Ground
  Ground_2 : Ground
  Ground_3 : Ground
  VISUCasingLights_Mux : Subsystem  Tag=mux/VisuCasingLights  mask(PreScan User Interface: VisuTrafficLight){}
      mask help:
      | The VisuTrafficLight block provides a way to animate traffic lights: switch on and off individual lights.
      |
      | For more information, please click Help.
      mask Help: eval('openHelp(731)')
  VISUCasingLights_TrafficLightRoadSideNL_4 : Outport  Tag=outport/VisuCasingLights  SampleTime=1/100
  wires:
  VISUCasingLights_Mux/1(VISUCasingLights_TrafficLightRoadSideNL_4) -> VISUCasingLights_TrafficLightRoadSideNL_4/1
  Ground_1/1 -> VISUCasingLights_Mux/1(Green [-])
  Ground_2/1 -> VISUCasingLights_Mux/2(Orange [-])
  Ground_3/1 -> VISUCasingLights_Mux/3(Red [-])

== system Base_Map_M_cs/TrafficLightRoadSideNL_5 ==
  Ground_1 : Ground
  Ground_2 : Ground
  Ground_3 : Ground
  VISUCasingLights_Mux : Subsystem  Tag=mux/VisuCasingLights  mask(PreScan User Interface: VisuTrafficLight){}
      mask help:
      | The VisuTrafficLight block provides a way to animate traffic lights: switch on and off individual lights.
      |
      | For more information, please click Help.
      mask Help: eval('openHelp(731)')
  VISUCasingLights_TrafficLightRoadSideNL_5 : Outport  Tag=outport/VisuCasingLights  SampleTime=1/100
  wires:
  VISUCasingLights_Mux/1(VISUCasingLights_TrafficLightRoadSideNL_5) -> VISUCasingLights_TrafficLightRoadSideNL_5/1
  Ground_1/1 -> VISUCasingLights_Mux/1(Green [-])
  Ground_2/1 -> VISUCasingLights_Mux/2(Orange [-])
  Ground_3/1 -> VISUCasingLights_Mux/3(Red [-])
